simulink model "hw2_signal_q4_3_fixed"  (R2018b)
settings: Solver=VariableStepAuto  StartTime=0  StopTime=150  RelTol=1e-3
settings Model: Creator=Sazgar Shargh  LastModifiedBy=Sazgar Shargh

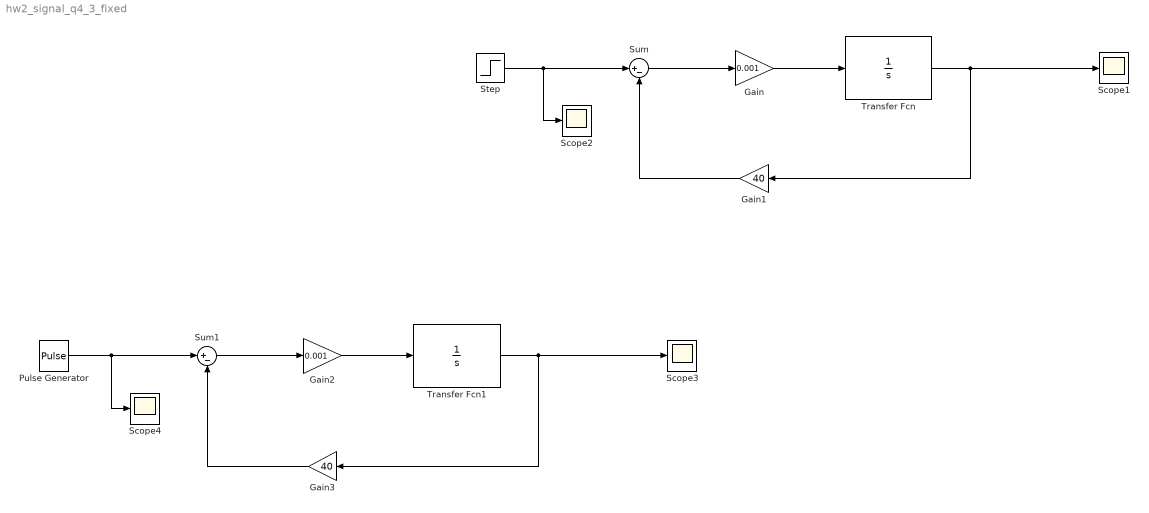
== system hw2_signal_q4_3_fixed ==
  Gain : Gain  Gain=0.001
  Gain1 : Gain  Gain=40
  Gain2 : Gain  Gain=0.001
  Gain3 : Gain  Gain=40
  Pulse Generator : DiscretePulseGenerator  PulseType=Time based  Amplitude=400  Period=200  PhaseDelay=10
  Scope{1..4} (4 alike) : Scope
  Step : Step  Time=0.0001  After=500  SampleTime=5
  Sum : Sum  Inputs=|+-
  Sum1 : Sum  Inputs=|+-
  Transfer Fcn : TransferFcn  Denominator=[1 0]
  Transfer Fcn1 : TransferFcn  Denominator=[1 0]
  wires:
  Step/1 -> Scope2/1, Sum/1
  Gain/1 -> Transfer Fcn/1
  Transfer Fcn/1 -> Gain1/1, Scope1/1
  Sum/1 -> Gain/1
  Gain1/1 -> Sum/2
  Transfer Fcn1/1 -> Gain3/1, Scope3/1
  Sum1/1 -> Gain2/1
  Pulse Generator/1 -> Scope4/1, Sum1/1
  Gain3/1 -> Sum1/2
  Gain2/1 -> Transfer Fcn1/1
